simulink model "tclab_model (1)"  (R2026a)
settings: Solver=VariableStepAuto  StopTime=1000
values from neighbouring files (symbols this model uses):
  A = 1e-3    (= 0.001)    [p3_lab2_comparacao (1).m]    (also in p3_lab2_comparacao.m; tclabsim.m)
  alpha = 0.0131    [p3_lab2_comparacao (1).m]    (also in p3_lab2_comparacao.m; tclabsim.m = p(2))
  Cp = 500    [p3_lab2_comparacao (1).m]    (also in p3_lab2_comparacao.m; tclabsim.m)
  m = 0.004    [p3_lab2_comparacao (1).m]    (also in p3_lab2_comparacao.m; tclabsim.m)
  sigma = 5.67e-8    (= 5.67e-08)    [p3_lab2_comparacao (1).m]    (also in p3_lab2_comparacao.m; tclabsim.m)
  TA = TA_C + 273.15    [p3_lab2_comparacao (1).m]    (also in p3_lab2_comparacao.m; tclabsim.m)
  tau = 21.1    [p3_lab2_comparacao (1).m]    (also in p3_lab2_comparacao.m; tclabsim.m = p(3))
  U = 4.4    [p3_lab2_comparacao (1).m]    (also in p3_lab2_comparacao.m; tclabsim.m = p(1))
  x0 = TA    [p3_lab2_comparacao (1).m]    (also in p3_lab2_comparacao.m)
settings Model: Creator=acer  LastModifiedBy=acer
settings DataIOCC: ExternalInput=[t' , u(1,:)']

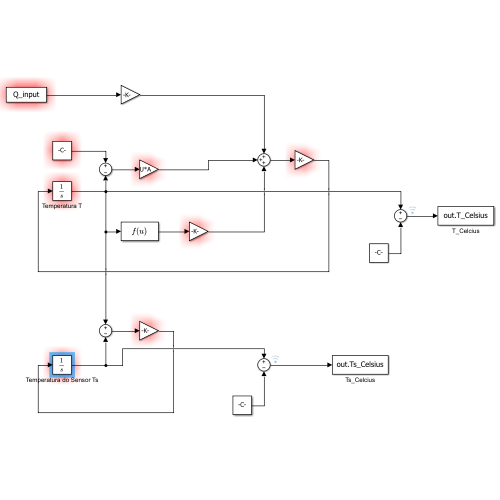
[thumbnail: Simulink's stored preview of the top-level diagram]
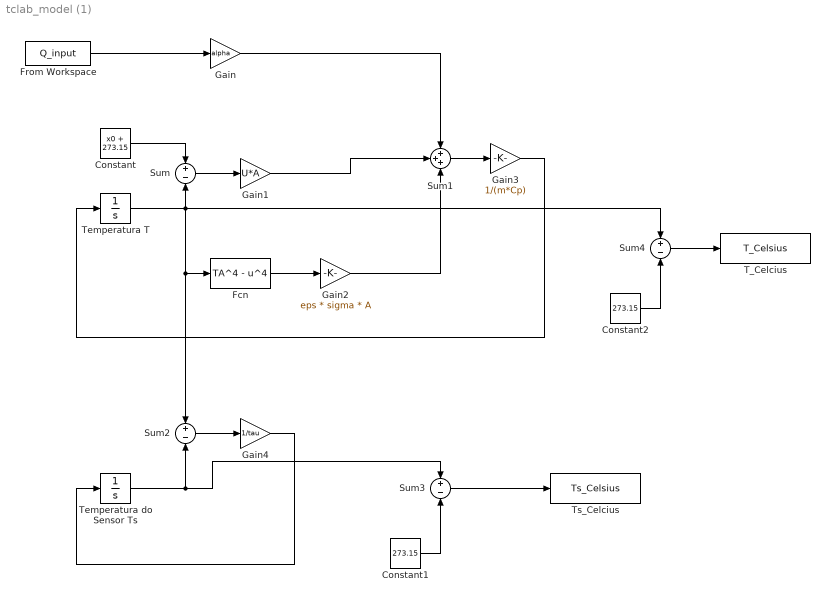
== system tclab_model (1) ==
  Constant : Constant  Value=x0 + 273.15
  Constant1 : Constant  Value=273.15
  Constant2 : Constant  Value=273.15
  Fcn : Fcn  Expr=TA^4 - u^4
  From Workspace : FromWorkspace  VariableName=Q_input
  Gain : Gain  Gain=alpha
  Gain1 : Gain  Gain=U*A
  Gain2 : Gain  Gain=eps * sigma * A
  Gain3 : Gain  Gain=1/(m*Cp)
  Gain4 : Gain  Gain=1/tau
  Sum{,2..4} (4 alike) : Sum  Inputs=+-
  Sum1 : Sum  Inputs=+++
  T_Celcius : ToWorkspace  VariableName=T_Celsius  SaveFormat=Timeseries  SampleTime=-1
  Temperatura T : Integrator  InitialCondition=x0 + 273.15
  Temperatura do Sensor Ts : Integrator  InitialCondition=x0 + 273.15
  Ts_Celcius : ToWorkspace  VariableName=Ts_Celsius  SaveFormat=Timeseries  SampleTime=-1
  wires:
  From Workspace/1 -> Gain/1
  Constant/1 -> Sum/1
  Temperatura T/1 -> Sum4/1, Sum/2, Sum2/1, Fcn/1
  Sum/1 -> Gain1/1
  Fcn/1 -> Gain2/1
  Gain/1 -> Sum1/1
  Gain1/1 -> Sum1/2
  Gain2/1 -> Sum1/3
  Sum1/1 -> Gain3/1
  Gain3/1 -> Temperatura T/1
  Temperatura do Sensor Ts/1 -> Sum3/1, Sum2/2
  Sum2/1 -> Gain4/1
  Gain4/1 -> Temperatura do Sensor Ts/1
  Constant1/1 -> Sum3/2
  Constant2/1 -> Sum4/2
  Sum4/1 -> T_Celcius/1
  Sum3/1 -> Ts_Celcius/1
